simulink model "testHarness"  (R2025a)
settings: Solver=VariableStepAuto  StartTime=0.0  StopTime=50  FixedStep=0.002  RelTol=1e-3  EnableMultiTasking=on
libraries: simulink x1
settings Model: ExtModeTrigDuration=10000  Creator=jellu  LastModifiedBy=Ayush_S
settings SolverCC: AlgebraicLoopSolver=TrustRegion  PositivePriorityOrder=on
settings DataIOCC: ReturnWorkspaceOutputs=off
settings OptimizationCC: LifeSpan=inf
settings DebuggingCC: UnconnectedInputMsg=warning  UnconnectedOutputMsg=warning  UnconnectedLineMsg=warning  ArithmeticOperatorsInVariantConditions=warning
settings ModelReferenceCC: EnableRefExpFcnMdlSchedulingChecks=on
settings SFSimCC: SimUseLocalCustomCode=off  CustomCodeUndefinedFunction=UseInterfaceOnly
settings RTWCC: SystemTargetFile=quarc_win64.tlc  TemplateMakefile=quarc_default_tmf  RTWUseLocalCustomCode=off  GPUComputeCapability=3.5  Description=QUARC Win64 Target
settings CodeAppCC: StateflowObjectComments=on
settings STFCustomTargetCC: SystemTargetFile=quarc_win64.tlc  TargetPreCompLibLocation=C:\PROGRA~3\QUARC\lib\2016a\win64\release  TargetLangStandard=C99 (ISO)  MultiwordLength=2048.0  DynamicStringBufferSize=256.0  ConcurrentExecutionCompliant=on  DownloadToTarget=on  StopOnOverrun=off  Debug=off
settings GRTTargetCC: ExtMode=on  ExtModeMexFile=quarc_comm  TargetPreCompLibLocation=C:\PROGRA~3\QUARC\lib\2016a\win64\release  ParMdlRefBuildCompliant=off  CompOptLevelCompliant=off  CombineOutputUpdateFcns=off  MatFileLogging=off  CPPClassGenCompliant=off  GRTInterface=on  UseToolchainInfoCompliant=off
settings ConfigComp: CovMetricSettings=dswe

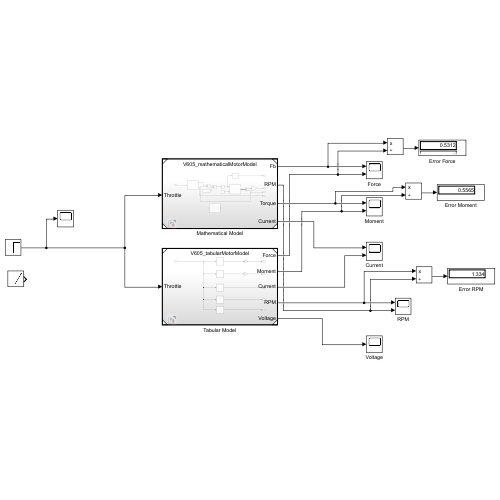
[thumbnail: Simulink's stored preview of the top-level diagram]
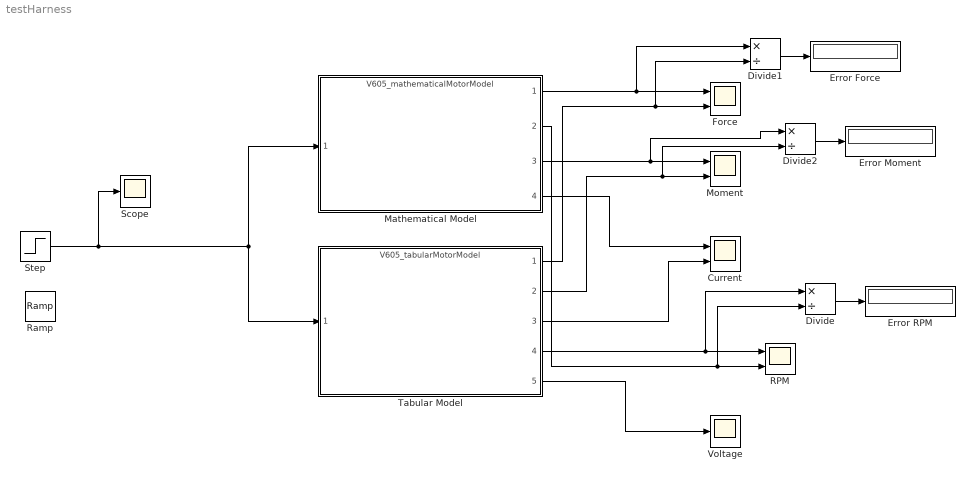
== system testHarness ==
  Current : Scope  NumInputPorts=2
      settings: ActiveDisplayYMinimum=-179.29366920011802  ActiveDisplayYMaximum=380.96953861017818  DataLoggingVariableName=ScopeData2
  Divide : Product  Inputs=*/
  Divide1 : Product  Inputs=*/
  Divide2 : Product  Inputs=*/
  Error Force : Display
  Error Moment : Display
  Error RPM : Display
  Force : Scope  NumInputPorts=2
      settings: ActiveDisplayYMinimum=-76.95646714600835  ActiveDisplayYMaximum=170.03046147106213
  Mathematical Model : ModelReference  ModelNameDialog=V605_mathematicalMotorModel.slx  SimulationMode=Normal  ModelReferenceVersion=3.33
  Moment : Scope  NumInputPorts=2
      settings: ActiveDisplayYMinimum=-23.12374207937777  ActiveDisplayYMaximum=26.681959002216953
  RPM : Scope  NumInputPorts=2
      settings: ActiveDisplayYMinimum=-116424.2948201094  ActiveDisplayYMaximum=154386.17922601497  DataLoggingVariableName=ScopeData5
  Ramp : simulink/Sources/Ramp  slope=1  start=0  InitialOutput=0
  Scope : Scope
      settings: ActiveDisplayYMinimum=-1017.7572108954528  ActiveDisplayYMaximum=899.31407017255765  DataLoggingVariableName=ScopeData7
  Step : Step  Time=0  After=50  SampleTime=0
  Tabular Model : ModelReference  ModelNameDialog=V605_tabularMotorModel.slx  SimulationMode=Normal  ModelReferenceVersion=3.3
  Voltage : Scope
      settings: ActiveDisplayYMinimum=-60.0072513102038  ActiveDisplayYMaximum=152.31085406867371  DataLoggingVariableName=ScopeData4
  wires:
  Mathematical Model/4 -> Current/1
  Tabular Model/3 -> Current/2
  Tabular Model/5 -> Voltage/1
  Tabular Model/4 -> Divide/1, RPM/1
  Mathematical Model/1 -> Divide1/1, Force/1
  Mathematical Model/2 -> Divide/2, RPM/2
  Divide/1 -> Error RPM/1
  Step/1 -> Scope/1, Tabular Model/1, Mathematical Model/1
  Tabular Model/1 -> Force/2, Divide1/2
  Divide1/1 -> Error Force/1
  Mathematical Model/3 -> Divide2/1, Moment/1
  Tabular Model/2 -> Divide2/2, Moment/2
  Divide2/1 -> Error Moment/1
